simulink model "simulink_example_osqp"  (R2024b)
settings: Solver=ode4  StartTime=0.0  StopTime=100  FixedStep=0.01  RelTol=1e-3
settings Model: Creator=lxxu  LastModifiedBy=lxxu

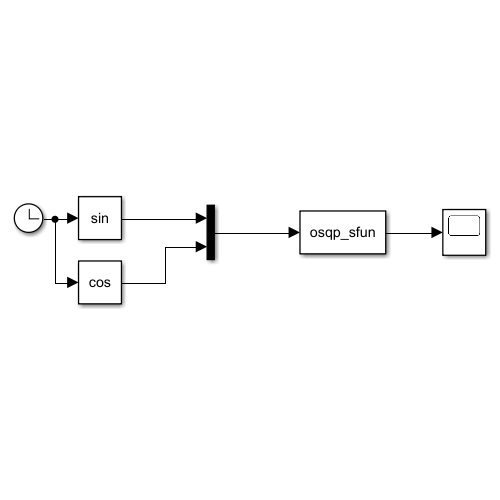
[thumbnail: Simulink's stored preview of the top-level diagram]
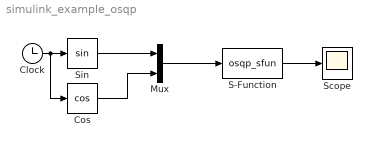
== system simulink_example_osqp ==
  Clock : Clock
  Cos : Trigonometry  Operator=cos
  Mux : Mux  Inputs=2
  S-Function : S-Function  FunctionName=osqp_sfun  SFunctionDeploymentMode=off  EnableBusSupport=off
  Scope : Scope
  Sin : Trigonometry
  wires:
  S-Function/1 -> Scope/1
  Clock/1 -> Cos/1, Sin/1
  Sin/1 -> Mux/1
  Cos/1 -> Mux/2
  Mux/1 -> S-Function/1
